simulink model "sldemo_tank1"  (Simulink 7.0)
settings: Solver=ode3  SolverMode=SingleTasking  StartTime=0.0  StopTime=400  FixedStep=.1  RelTol=1e-3  AbsTol=1e-6
PreLoadFcn:
  | sldemo_tankgui
StartFcn:
  | sldemo_tankgui start
StopFcn:
  | sldemo_tankgui stop
undefined symbols (not defined in the file or in its folder): area, hilim, inflow, lolim, outflow, sigbuilder_block
Description:
  | Tank Fill and Empty with Animation
  | 
  | This demonstration shows how to model the dynamics of liquid in a tank. The
  | associated animation provides a graphical display of the tank as it empties and
  | refills, based on user-defined tank parameters. The tank empties at the start
  | of the simulation and again part way through the simulation. When the simulation
  | is stopped, a plot is generated showing the liquid height and the states of the
  | two valves.
CloseFcn:
  | sldemo_tankgui done
settings Model: Creator=The MathWorks Inc.  LastModifiedBy=Amir  ExtModeTrigMode=oneshot  ExtModeArmWhenConnect=off  ExtModeAutoUpdateStatusClock=off
settings DataIOCC: LimitDataPoints=off  SignalLoggingName=sigsOut
settings OptimizationCC: InlineInvariantSignals=on  BufferReusableBoundary=off
settings DebuggingCC: SaveWithParameterizedLinksMsg=none  SignalResolutionControl=TryResolveAllWithWarning  SolverPrmCheckMsg=none  MultiTaskDSMMsg=warning  MultiTaskCondExecSysMsg=none  IntegerOverflowMsg=none  BusObjectLabelMismatch=none  StrictBusMsg=None
settings HardwareCC: TargetUnknown=on
settings RTWCC: IncludeERTFirstTime=on
settings CodeAppCC: CustomSymbolStrFcn=$F$N$M
settings GRTTargetCC: TargetFcnLib=ansi_tfl_tmw.mat

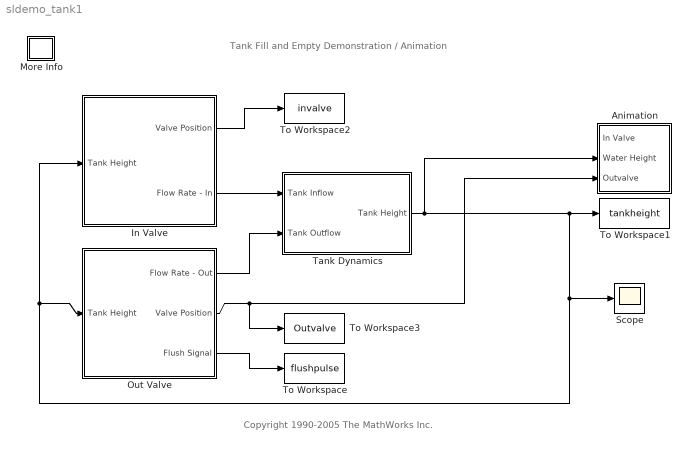
== system sldemo_tank1 ==
  note: Tank Fill and Empty Demonstration / Animation
  note: Copyright 1990-2005 The MathWorks Inc.
  Animation : Subsystem
      mask Display: disp('Animation\nControl')
  In Valve : Subsystem
  More Info : Subsystem
      settings: OpenFcn=showdemo(bdroot(gcs))
      mask Display: disp('?')
  Out Valve : Subsystem
  Scope : Scope
      settings: TickLabels=on  TimeRange=20  YMin=0  YMax=12.5  DataFormat=Array
  Tank Dynamics : Subsystem
  To Workspace : ToWorkspace  VariableName=flushpulse  SampleTime=-1  SaveFormat=Array
  To Workspace1 : ToWorkspace  VariableName=tankheight  SampleTime=-1  SaveFormat=Array
  To Workspace2 : ToWorkspace  VariableName=invalve  SampleTime=-1  SaveFormat=Array
  To Workspace3 : ToWorkspace  VariableName=Outvalve  SampleTime=-1  SaveFormat=Array
  wires:
  Out Valve/2(Valve Position) -> Animation/3(Outvalve), To Workspace3/1
  Tank Dynamics/1(Tank Height) -> Animation/2(Water Height), To Workspace1/1, Scope/1, Out Valve/1(Tank Height), In Valve/1(Tank Height)
  Out Valve/1(Flow Rate - Out) -> Tank Dynamics/2(Tank Outflow)
  Out Valve/3(Flush Signal) -> To Workspace/1
  In Valve/1(Valve Position) -> To Workspace2/1
  In Valve/2(Flow Rate - In) -> Tank Dynamics/1(Tank Inflow)

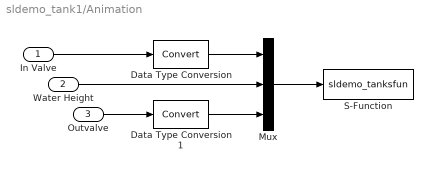
== system sldemo_tank1/Animation ==
  In Valve : Inport  OutDataType=sfix(16)  OutScaling=2^0
  Water Height : Inport  Port=2  OutDataType=sfix(16)  OutScaling=2^0
  Outvalve : Inport  Port=3  OutDataType=sfix(16)  OutScaling=2^0
  Data Type Conversion : DataTypeConversion  OutDataTypeMode=double  OutDataType=sfix(16)  OutScaling=2^0  SaturateOnIntegerOverflow=on  RndMeth=Zero
  Data Type Conversion1 : DataTypeConversion  OutDataTypeMode=double  OutDataType=sfix(16)  OutScaling=2^0  SaturateOnIntegerOverflow=on  RndMeth=Zero
  Mux : Mux  Inputs=3
  S-Function : S-Function  FunctionName=sldemo_tanksfun  Parameters=inflow,outflow,lolim,hilim,area
  wires:
  Outvalve/1 -> Data Type Conversion1/1
  Water Height/1 -> Mux/2
  Mux/1 -> S-Function/1
  In Valve/1 -> Data Type Conversion/1
  Data Type Conversion1/1 -> Mux/3
  Data Type Conversion/1 -> Mux/1

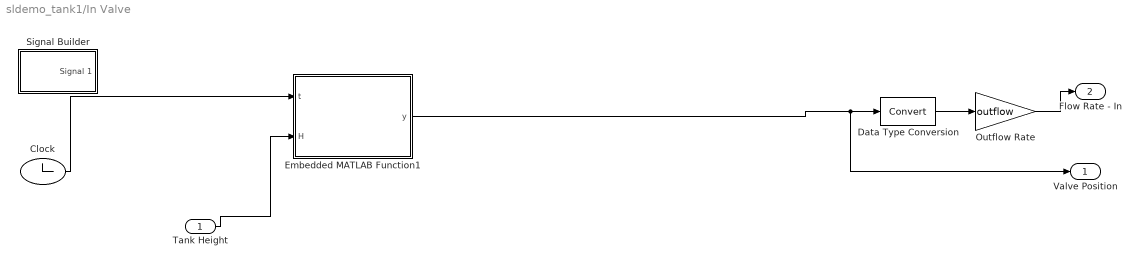
== system sldemo_tank1/In Valve ==
  Tank Height : Inport  OutDataType=sfix(16)  OutScaling=2^0
  Clock : Clock
      settings: Decimation=2
  Data Type Conversion : DataTypeConversion  OutDataTypeMode=double  OutDataType=sfix(16)  OutScaling=2^0  SaturateOnIntegerOverflow=on  RndMeth=Zero
  Embedded MATLAB Function1 : Stateflow chart
  Outflow Rate : Gain  Gain=outflow  ParameterDataType=sfix(16)  ParameterScaling=2^0  OutDataType=sfix(16)  OutScaling=2^0  SaturateOnIntegerOverflow=on
  Signal Builder : Subsystem  Tag=STV Subsys  LoadFcn=sigbuilder_block('load');  StartFcn=sigbuilder_block('start');  StopFcn=sigbuilder_block('stop');  ClipboardFcn=sigbuilder_block('clipboard');  mask(Sigbuilder block){}
      mask help: Sigbuilder GUI
      mask init:
      | if ~strcmp(get_param(bdroot(gcb),'SimulationStatus'),'stopped') tuvar = sigbuilder_block('maskInit'); end
      settings: CopyFcn=sigbuilder_block('copy');  DeleteFcn=sigbuilder_block('delete');  ModelCloseFcn=sigbuilder_block('modelClose');  PreSaveFcn=sigbuilder_block('preSave');  NameChangeFcn=sigbuilder_block('namechange');  OpenFcn=sigbuilder_block('open',[178.5 191.25 618.75 375 ]);  CloseFcn=sigbuilder_block('close');
      mask Display: plot(0,0,100,100,[10,10,40,40,10],[80,20,20,80,80],[40,10],[50,50], [40,27,10],[65,72,56],[40,25,25,10],[28,28,43,43]);
  Valve Position : Outport  OutDataType=sfix(16)  OutScaling=2^0  InitialOutput=0
  Flow Rate - In : Outport  Port=2  OutDataType=sfix(16)  OutScaling=2^0  InitialOutput=0
  wires:
  Tank Height/1 -> Embedded MATLAB Function1/2(H)
  Embedded MATLAB Function1/1(y) -> Valve Position/1, Data Type Conversion/1
  Outflow Rate/1 -> Flow Rate - In/1
  Data Type Conversion/1 -> Outflow Rate/1
  Clock/1 -> Embedded MATLAB Function1/1(t)

== system sldemo_tank1/More Info ==

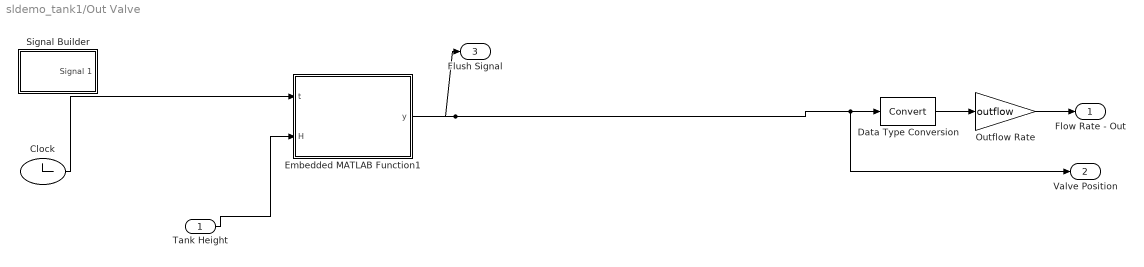
== system sldemo_tank1/Out Valve ==
  Tank Height : Inport  OutDataType=sfix(16)  OutScaling=2^0
  Clock : Clock
      settings: Decimation=2
  Data Type Conversion : DataTypeConversion  OutDataTypeMode=double  OutDataType=sfix(16)  OutScaling=2^0  SaturateOnIntegerOverflow=on  RndMeth=Zero
  Embedded MATLAB Function1 : Stateflow chart
  Outflow Rate : Gain  Gain=outflow  ParameterDataType=sfix(16)  ParameterScaling=2^0  OutDataType=sfix(16)  OutScaling=2^0  SaturateOnIntegerOverflow=on
  Signal Builder : Subsystem  Tag=STV Subsys  LoadFcn=sigbuilder_block('load');  StartFcn=sigbuilder_block('start');  StopFcn=sigbuilder_block('stop');  ClipboardFcn=sigbuilder_block('clipboard');  mask(Sigbuilder block){}
      mask help: Sigbuilder GUI
      mask init:
      | if ~strcmp(get_param(bdroot(gcb),'SimulationStatus'),'stopped') tuvar = sigbuilder_block('maskInit'); end
      settings: CopyFcn=sigbuilder_block('copy');  DeleteFcn=sigbuilder_block('delete');  ModelCloseFcn=sigbuilder_block('modelClose');  PreSaveFcn=sigbuilder_block('preSave');  NameChangeFcn=sigbuilder_block('namechange');  OpenFcn=sigbuilder_block('open',[178.5 191.25 618.75 375 ]);  CloseFcn=sigbuilder_block('close');
      mask Display: plot(0,0,100,100,[10,10,40,40,10],[80,20,20,80,80],[40,10],[50,50], [40,27,10],[65,72,56],[40,25,25,10],[28,28,43,43]);
  Flow Rate - Out : Outport  OutDataType=sfix(16)  OutScaling=2^0  InitialOutput=0
  Valve Position : Outport  Port=2  OutDataType=sfix(16)  OutScaling=2^0  InitialOutput=0
  Flush Signal : Outport  Port=3  OutDataType=sfix(16)  OutScaling=2^0  InitialOutput=0
  wires:
  Tank Height/1 -> Embedded MATLAB Function1/2(H)
  Embedded MATLAB Function1/1(y) -> Valve Position/1, Data Type Conversion/1, Flush Signal/1
  Outflow Rate/1 -> Flow Rate - Out/1
  Data Type Conversion/1 -> Outflow Rate/1
  Clock/1 -> Embedded MATLAB Function1/1(t)

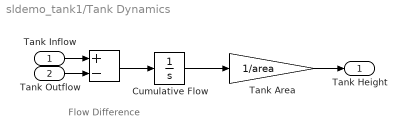
== system sldemo_tank1/Tank Dynamics ==
  note: Flow
      | Difference
  Tank Inflow : Inport  OutDataType=sfix(16)  OutScaling=2^0
  Tank Outflow : Inport  Port=2  OutDataType=sfix(16)  OutScaling=2^0
  " " : Sum  Inputs=+-  OutDataType=sfix(16)  OutScaling=2^0  SaturateOnIntegerOverflow=on  InputSameDT=on
  Cumulative Flow : Integrator  InitialCondition=(hilim+lolim)/2*area
  Tank Area : Gain  Gain=1/area  ParameterDataType=sfix(16)  ParameterScaling=2^0  OutDataType=sfix(16)  OutScaling=2^0  SaturateOnIntegerOverflow=on
  Tank Height : Outport  OutDataType=sfix(16)  OutScaling=2^0  InitialOutput=0
  wires:
  Tank Outflow/1 -> " "/2
  Tank Inflow/1 -> " "/1
  " "/1 -> Cumulative Flow/1
  Cumulative Flow/1 -> Tank Area/1
  Tank Area/1 -> Tank Height/1

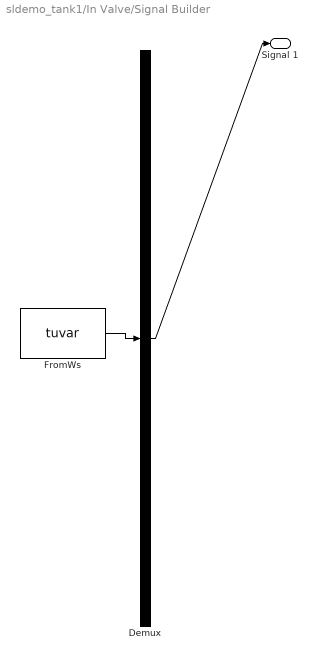
== system sldemo_tank1/In Valve/Signal Builder ==
  Demux : Demux  Tag=STV Demux  Outputs=1
  FromWs : FromWorkspace  Tag=STV FromWs  VariableName=tuvar  SampleTime=0  SigBuilderData=DataTag0  VnvData=DataTag1
      SigBuilderData=|
      | channels.label = 'Signal 1'
      | channels.allXData = {[0 40.2 40.2 90 90 150]}
      | channels.allYData = {[0 0 1 1 0 0]}
      | dataSet.timeRange = [0 150]
      | dataSet.name = 'Group 1'
  Signal 1 : Outport  Tag=STV Outport
  wires:
  FromWs/1 -> Demux/1
  Demux/1 -> Signal 1/1

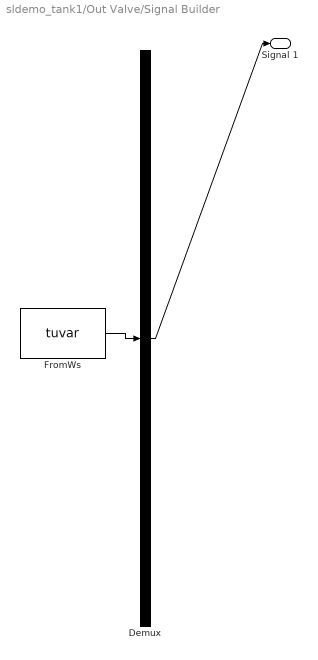
== system sldemo_tank1/Out Valve/Signal Builder ==
  Demux : Demux  Tag=STV Demux  Outputs=1
  FromWs : FromWorkspace  Tag=STV FromWs  VariableName=tuvar  SampleTime=0  SigBuilderData=DataTag2  VnvData=DataTag3
      SigBuilderData=|
      | channels.label = 'Signal 1'
      | channels.allXData = {[0 40.2 40.2 90 90 150]}
      | channels.allYData = {[0 0 1 1 0 0]}
      | dataSet.timeRange = [0 150]
      | dataSet.name = 'Group 1'
  Signal 1 : Outport  Tag=STV Outport
  wires:
  FromWs/1 -> Demux/1
  Demux/1 -> Signal 1/1

== matlab function Out Valve/Embedded MATLAB Function1 ==
  data: y output double; t input inherited; H input inherited
function y = timeavg(t,H)
%TIMEAVG Compute time average of input signal U.
%   Y = TIMEAVG(U,T) computes the time average of U,
%   where T is the current simulation time.


% Declare variables that must retain values between iterations.

persistent last_y last_t T1 T2;
lam1=0.3; %On parameter
lam2=1; %Off parameter
N =3; % number of PUs

% Initialize persistent variables in the first iteration.
if isempty(last_t)
   disp(['initialize'])
   last_y = zeros(N,1);
  
   last_t = zeros(N,1);
   T1=zeros(N,1); % ON time
   T2=zeros(N,1); % OFF Time
   
   T1=random('exponential',lam1,N,1);
   T1=random('exponential',lam1,N,1);
   
end
y=sum(last_y);

delta=t*ones(N,1)-last_t;

%disp(['t= ',num2str(t),', last_t= ',num2str(last_t),', delta= ',num2str(delta),', T1= ', num2str(T1),', y= ',num2str(y)...
%    ,', delta > T1= ',num2str(delta > T1)])

% Compute the outputs.
for i=1:N
    if (delta(i) > T1(i)) && (last_y(i)==1) % One PU turns off
       y = y-1; 
       last_y(i)=0;
       T1(i)=random('exponential',lam1);
       last_t(i) = t;
%       disp(['Turining OFF'])
    end
    
    if (delta(i) > T2(i)) && (last_y(i)==0) % One PU turns on
       y = y+1; 
       last_y(i)=1;
       T2(i)=random('exponential',lam1);
       last_t(i) = t;
%       disp(['Turining ON'])
    end
end

== matlab function In Valve/Embedded MATLAB Function1 ==
  data: y output double; t input inherited; H input inherited
function y = timeavg(t,H)
%TIMEAVG Compute time average of input signal U.
%   Y = TIMEAVG(U,T) computes the time average of U,
%   where T is the current simulation time.


hilim = 10000; % hilimit
% Declare variables that must retain values between iterations.
persistent last_y last_t T1 T2;
lam1=5; %On parameter
lam2=1; %Off parameter
N =5; % number of SUs

% Initialize persistent variables in the first iteration.
if isempty(last_t)
   disp(['initialize'])
   last_y = zeros(N,1);
  
   last_t = zeros(N,1);
   T1=zeros(N,1); % ON time
   T2=zeros(N,1); % OFF Time
   
   T1=random('exponential',lam1,N,1);
   T2=random('exponential',lam1,N,1);
   
end
y=sum(last_y);

delta=t*ones(N,1)-last_t;

%disp(['t= ',num2str(t),', last_t= ',num2str(last_t),', delta= ',num2str(delta),', T1= ', num2str(T1),', y= ',num2str(y)...
%    ,', delta > T1= ',num2str(delta > T1)])

% Compute the outputs.
if H<hilim
    for i=1:N
        if (delta(i) > T1(i)) && (last_y(i)==1) % One PU turns off
           y = y-1; 
           last_y(i)=0;
           T1(i)=random('exponential',lam1);
           last_t(i) = t;
          % disp(['Turining OFF'])
        end

        if (delta(i) > T2(i)) && (last_y(i)==0) % One PU turns on
           y = y+1; 
           last_y(i)=1;
           T2(i)=random('exponential',lam1);
           last_t(i) = t;
          % disp(['Turining ON'])
        end
    end
else
    y=0;
    last_y=zeros(N,1);
end
